simulink model "model_autopilot"  (R2019a)
settings: Solver=VariableStepAuto  StartTime=0.0  StopTime=sim_time  RelTol=1e-3
values from neighbouring files (symbols this model uses):
  a_phi_1 = -0.65    [A2_Part1.m]    (also in A2_Part1_e.m = 2.87)
  a_phi_2 = 2.87    [A2_Part1.m]    (also in A2_Part1_e.m = -0.65)
  d = 1.5    [A2_Part1.m]    (also in A2_Part1_e.m = 0.0261799387799)
  g = 9.81    [A2_model.m]
  k_d_phi = 0    [A2_Part1.m]    (also in A2_Part1_e.m = (2 * zeta_phi * omega_n_phi - a_phi_1)/a_phi_2)
  k_i_chi = 0    [A2_Part1.m]    (also in A2_Part1_e.m = omega_n_chi^2 * V_g/g)
  k_i_phi = 0    [A2_Part1.m]    (also in A2_Part1_e.m)
  k_p_chi = 0    [A2_Part1.m]    (also in A2_Part1_e.m = 2 * zeta_chi * omega_n_chi * V_g/g)
  k_p_phi = 0    [A2_Part1.m]    (also in A2_Part1_e.m = delta_a_max/e_phi_max * sign(a_phi_2))
  V_g = V_a    [A2_Part1.m]    (also in A2_Part1_e.m)
settings Model: Creator=gustavoo  LastModifiedBy=gustavoo

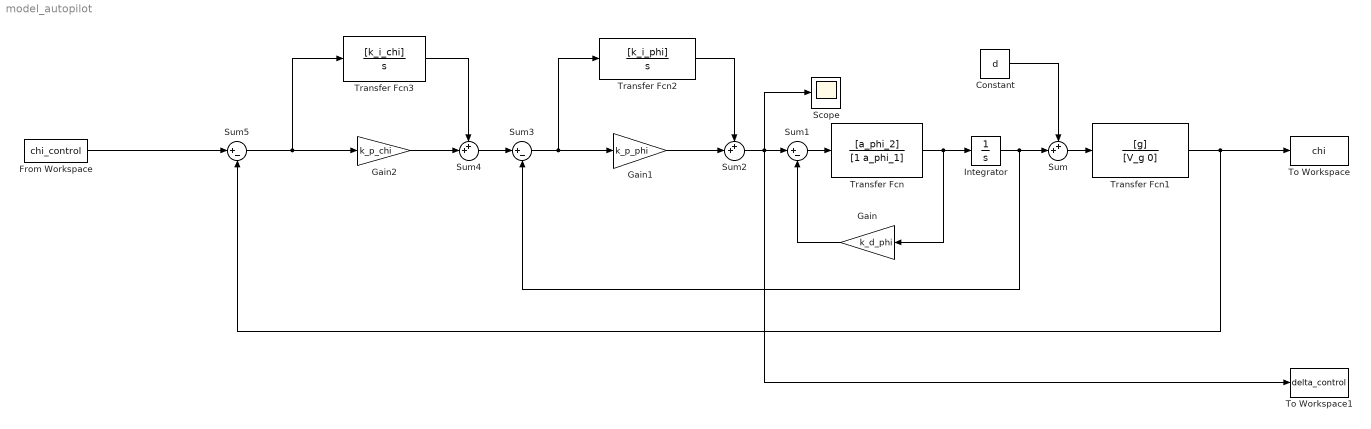
== system model_autopilot ==
  Constant : Constant  Value=d
  From Workspace : FromWorkspace  VariableName=chi_control  SampleTime=0
  Gain : Gain  Gain=k_d_phi
  Gain1 : Gain  Gain=k_p_phi
  Gain2 : Gain  Gain=k_p_chi
  Integrator : Integrator
  Scope : Scope
  Sum : Sum  Inputs=++|
  Sum1 : Sum  Inputs=|+-
  Sum2 : Sum  Inputs=++|
  Sum3 : Sum  Inputs=|+-
  Sum4 : Sum  Inputs=++|
  Sum5 : Sum  Inputs=|+-
  To Workspace : ToWorkspace  VariableName=chi  SaveFormat=Timeseries  SampleTime=-1
  To Workspace1 : ToWorkspace  VariableName=delta_control  SaveFormat=Timeseries  SampleTime=-1
  Transfer Fcn : TransferFcn  Numerator=[a_phi_2]  Denominator=[1 a_phi_1]
  Transfer Fcn1 : TransferFcn  Numerator=[g]  Denominator=[V_g 0]
  Transfer Fcn2 : TransferFcn  Numerator=[k_i_phi]  Denominator=[1 0]
  Transfer Fcn3 : TransferFcn  Numerator=[k_i_chi]  Denominator=[1 0]
  wires:
  Sum/1 -> Transfer Fcn1/1
  Integrator/1 -> Sum3/2, Sum/2
  Constant/1 -> Sum/1
  Transfer Fcn/1 -> Integrator/1, Gain/1
  Sum1/1 -> Transfer Fcn/1
  Gain/1 -> Sum1/2
  Sum2/1 -> Scope/1, To Workspace1/1, Sum1/1
  Transfer Fcn2/1 -> Sum2/1
  Gain1/1 -> Sum2/2
  Sum3/1 -> Transfer Fcn2/1, Gain1/1
  Sum4/1 -> Sum3/1
  Gain2/1 -> Sum4/2
  Transfer Fcn3/1 -> Sum4/1
  Sum5/1 -> Transfer Fcn3/1, Gain2/1
  Transfer Fcn1/1 -> To Workspace/1, Sum5/2
  From Workspace/1 -> Sum5/1
